simulink model "AGTF30SysDyn"  (Simulink 8.5)
settings: Solver=ode4  StartTime=0.0  StopTime=MWS.In.t(end)  FixedStep=MWS.In.Ts  RelTol=1e-3
model workspace: external: MAT-File (data not in the file)
values from neighbouring files (symbols this model uses):
  MWS = setup_InputsSS(MWS)    [define_inputs.m]
libraries: Lib_Cntrl_FirstOrderSensor_TMATS x12, Lib_Solve_ModelSource_TMATS x8, Lib_Cntrl_LimitCntrlPI_TMATS x5, Lib_Cntrl_FirstOrderActuator_TMATS x2, Lib_Cntrl_SetPoint_TMATS x2, Lib_Solve_OuterLoopIntegrator_TMATS x2, simulink x2, Lib_Cntrl_CorrectedSpeed_TMATS x1, Lib_Cntrl_LimitSelect_TMATS x1, Lib_Cntrl_SetPointCntrlPI_TMATS x1, Lib_Solve_IterNRSolverJC_TMATS x1
settings Model: Creator=jwchapm2  LastModifiedBy=jwchapm2
settings DataIOCC: SignalLoggingSaveFormat=Dataset
settings OptimizationCC: ExpressionDepthLimit=128
settings DebuggingCC: UnderspecifiedInitializationDetection=Simplified  MergeDetectMultiDrivingBlocksExec=error  FcnCallInpInsideContextMsg=EnableAllAsError  StateNameClashWarn=none
settings GRTTargetCC: CombineOutputUpdateFcns=on  GRTInterface=off

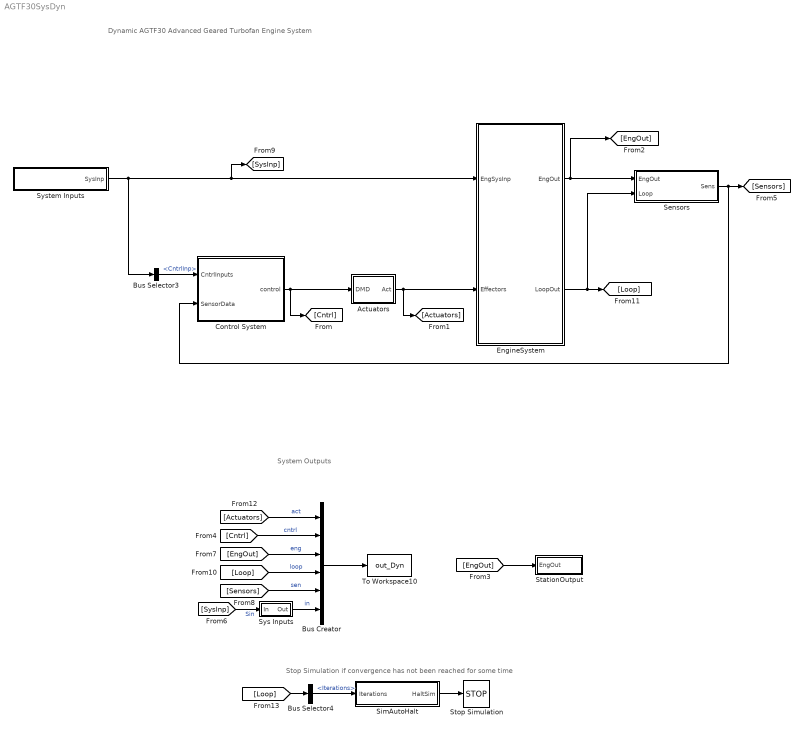
== system AGTF30SysDyn ==
  note: Stop Simulation if convergence has not been reached for some time
  note: Dynamic AGTF30
      | Advanced Geared Turbofan Engine System
  note: System Outputs
  Actuators : Subsystem
  Bus Creator : BusCreator  Inputs=6
  Bus Selector3 : BusSelector  OutputSignals=CntrlInp
  Bus Selector4 : BusSelector  OutputSignals=Solver.Iterations
  Control System : Subsystem
  EngineSystem : Subsystem
  Sensors : Subsystem
  SimAutoHalt : Subsystem
  StationOutput : Subsystem
  Stop Simulation : Stop
  Sys Inputs : Subsystem
  System Inputs : Subsystem
  To Workspace10 : ToWorkspace  VariableName=out_Dyn  SaveFormat=Timeseries  SampleTime=-1
  wires:
  Actuators/1(Act) -> [Actuators], EngineSystem/2(Effectors)
  Control System/1(control) -> Actuators/1(DMD), [Cntrl]
  Bus Selector3/1 -> Control System/1(CntrlInputs)  "<CntrlInp>"
  System Inputs/1(SysInp) -> Bus Selector3/1, EngineSystem/1(EngSysInp), [SysInp]
  EngineSystem/1(EngOut) -> [EngOut], Sensors/1(EngOut)
  EngineSystem/2(LoopOut) -> Sensors/2(Loop), [Loop]
  [EngOut] -> StationOutput/1(EngOut)
  Bus Creator/1 -> To Workspace10/1
  [Loop] -> Bus Creator/4  "loop"
  [Sensors] -> Bus Creator/5  "sen"
  [EngOut] -> Bus Creator/3  "eng"
  Sys Inputs/1(Out) -> Bus Creator/6  "in"
  [Actuators] -> Bus Creator/1  "act"
  [Cntrl] -> Bus Creator/2  "cntrl"
  Sensors/1(Sens) -> Control System/2(SensorData), [Sensors]
  [Loop] -> Bus Selector4/1
  Bus Selector4/1 -> SimAutoHalt/1(Iterations)  "<Iterations>"
  SimAutoHalt/1(HaltSim) -> Stop Simulation/1
  [SysInp] -> Sys Inputs/1(In)  "Sin"

== system AGTF30SysDyn/Actuators ==
  DMD : Inport
  Bus Creator : BusCreator  Inputs=3
  Bus Selector1 : BusSelector  OutputSignals=Wfdmd,VBVdmd,VAFNdmd
  FMV : Subsystem
  VAFN : Subsystem
  VBV : Subsystem
  Act : Outport
  wires:
  DMD/1 -> Bus Selector1/1
  Bus Creator/1 -> Act/1  "Actuator"
  Bus Selector1/3 -> VAFN/1(VAFNdmd)  "<VAFNdmd>"
  Bus Selector1/2 -> VBV/1(VBVdmd)  "<VBVdmd>"
  VBV/1(VBVact) -> Bus Creator/2  "VBVact"
  VAFN/1(VAFNact) -> Bus Creator/3  "VAFNact"
  Bus Selector1/1 -> FMV/1(Wfdmd)  "<Wfdmd>"
  FMV/1(Wfact) -> Bus Creator/1  "Wfact"

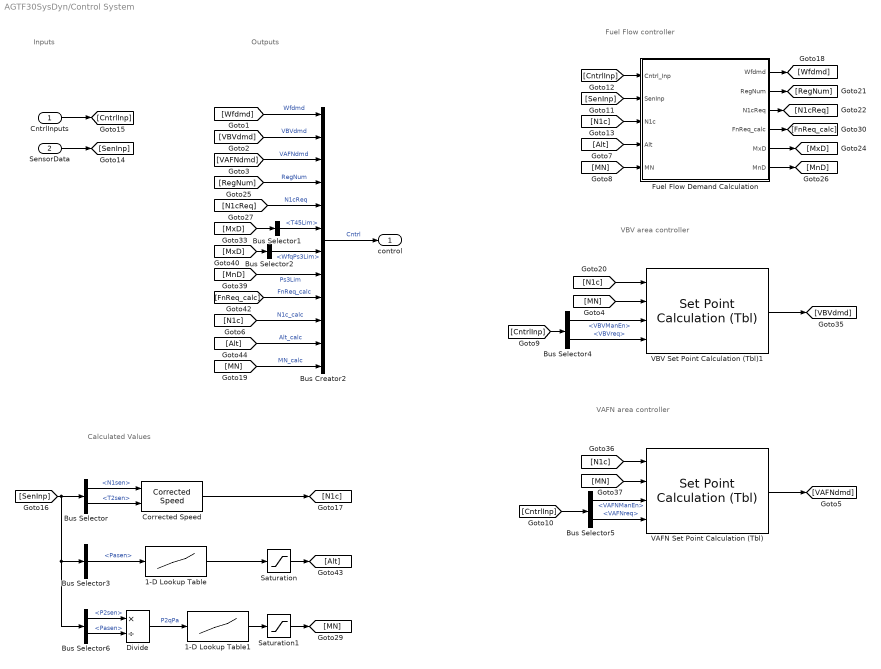
== system AGTF30SysDyn/Control System ==
  note: Inputs
  note: VAFN area controller
  note: VBV area controller
  note: Fuel Flow controller
  note: Calculated Values
  note: Outputs
  CntrlInputs : Inport
  SensorData : Inport  Port=2
  1-D Lookup Table : Lookup_n-D  NumberOfTableDimensions=1  BreakpointsForDimension1=MWS.Cntrl.AltCalc_PaVec  Table=MWS.Cntrl.AltCalc_AltVec  InternalRulePriority=Speed  RndMeth=Simplest  InputSameDT=on
  1-D Lookup Table1 : Lookup_n-D  NumberOfTableDimensions=1  BreakpointsForDimension1=MWS.Cntrl.MNCalc_P2qPa  Table=MWS.Cntrl.MNCalc_MNVec  InternalRulePriority=Speed  RndMeth=Simplest  InputSameDT=on
  Bus Creator2 : BusCreator  Inputs=12
  Bus Selector : BusSelector  OutputSignals=N.N1sen,T.T2sen
  Bus Selector1 : BusSelector  OutputSignals=T45Lim
  Bus Selector2 : BusSelector  OutputSignals=WfqPs3Lim
  Bus Selector3 : BusSelector  OutputSignals=P.Pasen
  Bus Selector4 : BusSelector  OutputSignals=ManualOp.VBVManEn,ManualOp.VBVreq
  Bus Selector5 : BusSelector  OutputSignals=ManualOp.VAFNManEn,ManualOp.VAFNreq
  Bus Selector6 : BusSelector  OutputSignals=P.P2sen,P.Pasen
  Corrected Speed : Lib_Cntrl_CorrectedSpeed_TMATS/Corrected Speed  C_TSTD_M=518.67
  Divide : Product  Inputs=*/
  Fuel Flow Demand Calculation : Subsystem
  Saturation : Saturate  UpperLimit=MWS.Cntrl.AltCalc_Altmax  LowerLimit=MWS.Cntrl.AltCalc_Altmin
  Saturation1 : Saturate  UpperLimit=MWS.Cntrl.MNCalc_MNmax  LowerLimit=MWS.Cntrl.MNCalc_MNmin
  VAFN Set Point Calculation (Tbl) : Lib_Cntrl_SetPoint_TMATS/Set Point Calculation (Tbl)  ERVec_M=MWS.Cntrl.VAFN_Nc1  DSVec_M=MWS.Cntrl.VAFN_MN  SPArray_M=MWS.Cntrl.VAFN_sch
  VBV Set Point Calculation (Tbl)1 : Lib_Cntrl_SetPoint_TMATS/Set Point Calculation (Tbl)  ERVec_M=MWS.Cntrl.VBV_Nc1  DSVec_M=MWS.Cntrl.VBV_MN  SPArray_M=MWS.Cntrl.VBV_sch
  control : Outport
  wires:
  CntrlInputs/1 -> [CntrlInp]
  [Wfdmd] -> Bus Creator2/1  "Wfdmd"
  [VBVdmd] -> Bus Creator2/2  "VBVdmd"
  [VAFNdmd] -> Bus Creator2/3  "VAFNdmd"
  SensorData/1 -> [SenInp]
  Bus Selector/1 -> Corrected Speed/1  "<N1sen>"
  Corrected Speed/1 -> [N1c]
  Bus Selector/2 -> Corrected Speed/2  "<T2sen>"
  [CntrlInp] -> Bus Selector4/1
  [RegNum] -> Bus Creator2/4  "RegNum"
  VAFN Set Point Calculation (Tbl)/1 -> [VAFNdmd]
  [CntrlInp] -> Bus Selector5/1
  Bus Selector4/1 -> VBV Set Point Calculation (Tbl)1/3  "<VBVManEn>"
  Bus Selector4/2 -> VBV Set Point Calculation (Tbl)1/4  "<VBVreq>"
  [MN] -> VBV Set Point Calculation (Tbl)1/2
  VBV Set Point Calculation (Tbl)1/1 -> [VBVdmd]
  Bus Selector5/2 -> VAFN Set Point Calculation (Tbl)/4  "<VAFNreq>"
  Bus Selector5/1 -> VAFN Set Point Calculation (Tbl)/3  "<VAFNManEn>"
  [MN] -> VAFN Set Point Calculation (Tbl)/2
  [N1c] -> VAFN Set Point Calculation (Tbl)/1
  [N1c] -> VBV Set Point Calculation (Tbl)1/1
  [N1c] -> Bus Creator2/10  "N1c_calc"
  [N1cReq] -> Bus Creator2/5  "N1cReq"
  Bus Selector1/1 -> Bus Creator2/6  "<T45Lim>"
  [MxD] -> Bus Selector1/1
  [MnD] -> Bus Creator2/8  "Ps3Lim"
  [MxD] -> Bus Selector2/1
  Bus Selector2/1 -> Bus Creator2/7  "<WfqPs3Lim>"
  [FnReq_calc] -> Bus Creator2/9  "FnReq_calc"
  1-D Lookup Table/1 -> Saturation/1
  [SenInp] -> Bus Selector6/1, Bus Selector3/1, Bus Selector/1
  Bus Selector3/1 -> 1-D Lookup Table/1  "<Pasen>"
  Bus Selector6/1 -> Divide/1  "<P2sen>"
  Bus Selector6/2 -> Divide/2  "<Pasen>"
  Divide/1 -> 1-D Lookup Table1/1  "P2qPa"
  1-D Lookup Table1/1 -> Saturation1/1
  [Alt] -> Bus Creator2/11  "Alt_calc"
  [MN] -> Bus Creator2/12  "MN_calc"
  Saturation/1 -> [Alt]
  Saturation1/1 -> [MN]
  Bus Creator2/1 -> control/1  "Cntrl"
  [CntrlInp] -> Fuel Flow Demand Calculation/1(Cntrl_Inp)
  [Alt] -> Fuel Flow Demand Calculation/4("Alt ")
  [MN] -> Fuel Flow Demand Calculation/5(MN)
  [SenInp] -> Fuel Flow Demand Calculation/2(SenInp)
  [N1c] -> Fuel Flow Demand Calculation/3(N1c)
  Fuel Flow Demand Calculation/6(MnD) -> [MnD]
  Fuel Flow Demand Calculation/5(MxD) -> [MxD]
  Fuel Flow Demand Calculation/4(FnReq_calc) -> [FnReq_calc]
  Fuel Flow Demand Calculation/3(N1cReq) -> [N1cReq]
  Fuel Flow Demand Calculation/2(RegNum) -> [RegNum]
  Fuel Flow Demand Calculation/1(Wfdmd) -> [Wfdmd]

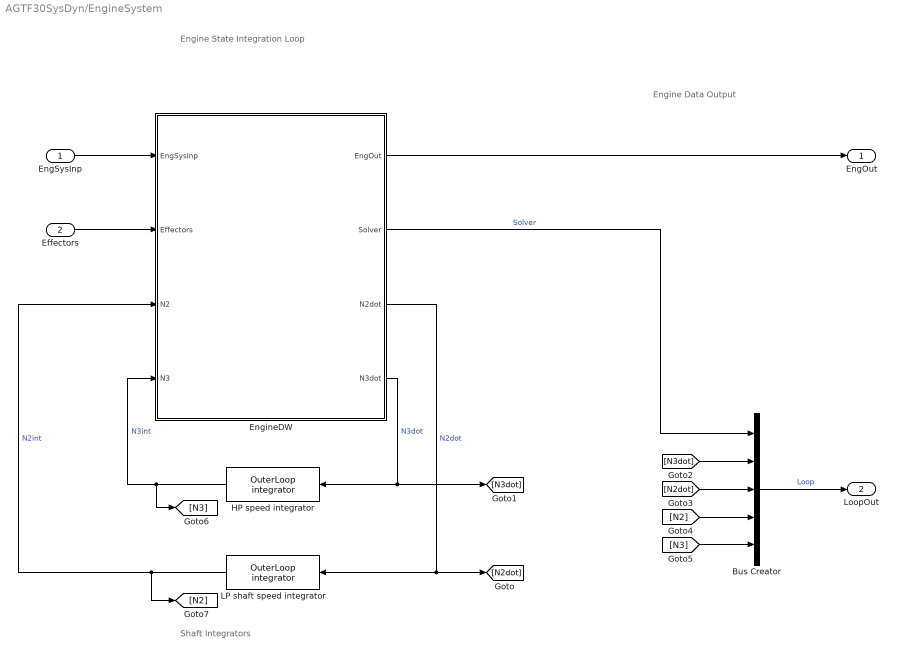
== system AGTF30SysDyn/EngineSystem ==
  note: Shaft Integrators
  note: Engine State
      | Integration Loop
  note: Engine Data Output
  EngSysInp : Inport
  Effectors : Inport  Port=2
  Bus Creator : BusCreator  Inputs=5
  EngineDW : Subsystem
  HP speed integrator : Lib_Solve_OuterLoopIntegrator_TMATS/OuterLoop integrator  OL_IC_M=MWS.In.N3IC
  LP shaft speed integrator : Lib_Solve_OuterLoopIntegrator_TMATS/OuterLoop integrator  OL_IC_M=MWS.In.N2IC
  EngOut : Outport
  LoopOut : Outport  Port=2
  wires:
  EngSysInp/1 -> EngineDW/1(EngSysInp)
  LP shaft speed integrator/1 -> [N2], EngineDW/3(N2)  "N2int"
  Effectors/1 -> EngineDW/2(Effectors)
  EngineDW/3(N2dot) -> LP shaft speed integrator/1, [N2dot]  "N2dot"
  EngineDW/2(Solver) -> Bus Creator/1  "Solver"
  EngineDW/1(EngOut) -> EngOut/1
  EngineDW/4(N3dot) -> HP speed integrator/1, [N3dot]  "N3dot"
  HP speed integrator/1 -> [N3], EngineDW/4(N3)  "N3int"
  Bus Creator/1 -> LoopOut/1  "Loop"
  [N3dot] -> Bus Creator/2
  [N2dot] -> Bus Creator/3
  [N2] -> Bus Creator/4
  [N3] -> Bus Creator/5

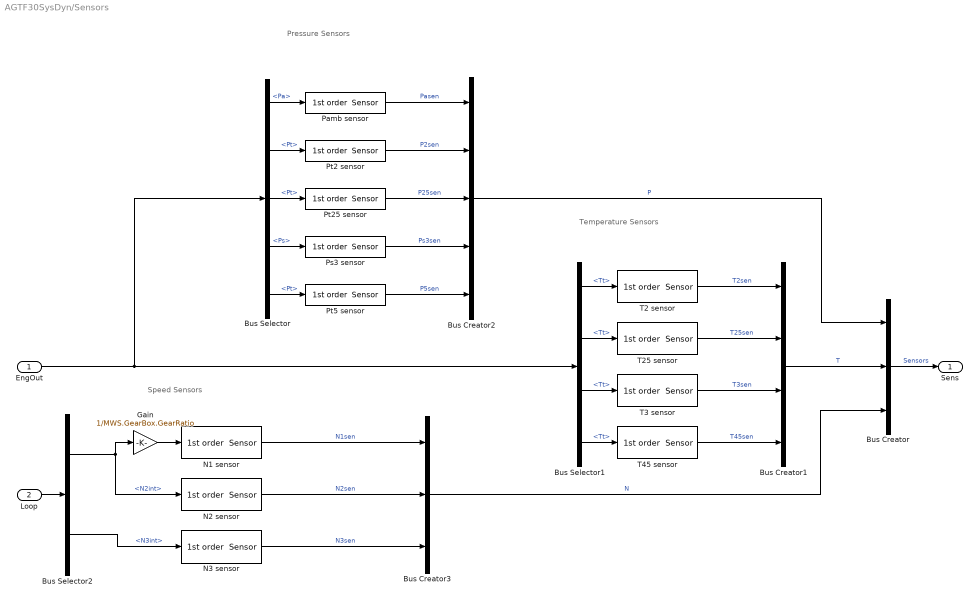
== system AGTF30SysDyn/Sensors ==
  note: Pressure Sensors
  note: Temperature Sensors
  note: Speed Sensors
  EngOut : Inport
  Loop : Inport  Port=2
  Bus Creator : BusCreator  Inputs=3
  Bus Creator1 : BusCreator
  Bus Creator2 : BusCreator  Inputs=5
  Bus Creator3 : BusCreator  Inputs=3
  Bus Selector : BusSelector  OutputSignals=Amb.Pa,S2.Pt,S25.Pt,S36.Ps,S5.Pt
  Bus Selector1 : BusSelector  OutputSignals=S2.Tt,S25.Tt,S36.Tt,S45.Tt
  Bus Selector2 : BusSelector  OutputSignals=N2int,N3int
  Gain : Gain  Gain=1/MWS.GearBox.GearRatio
  N1 sensor : Lib_Cntrl_FirstOrderSensor_TMATS/1st order  Sensor  IC_M=MWS.In.Sensor.ICN1  Sen_Max_M=MWS.Sensor.N1.Max  Sen_Min_M=MWS.Sensor.N1.Min  Gain_M=1  Tau_M=MWS.Sensor.N1.Tau  GN_EN_M=off  GN_NST_M=MWS.In.Ts  GN_C_M=1  GN_MinNoise_M=0.3  F_Gain_M=1  F_Drift_M=0
  N2 sensor : Lib_Cntrl_FirstOrderSensor_TMATS/1st order  Sensor  IC_M=MWS.In.Sensor.ICN2  Sen_Max_M=MWS.Sensor.N2.Max  Sen_Min_M=MWS.Sensor.N2.Min  Gain_M=1  Tau_M=MWS.Sensor.N2.Tau  GN_EN_M=off  GN_NST_M=MWS.In.Ts  GN_C_M=1  GN_MinNoise_M=0.3  F_Gain_M=1  F_Drift_M=0
  N3 sensor : Lib_Cntrl_FirstOrderSensor_TMATS/1st order  Sensor  IC_M=MWS.In.Sensor.ICN3  Sen_Max_M=MWS.Sensor.N3.Max  Sen_Min_M=MWS.Sensor.N3.Min  Gain_M=1  Tau_M=MWS.Sensor.N3.Tau  GN_EN_M=off  GN_NST_M=MWS.In.Ts  GN_C_M=1  GN_MinNoise_M=0.3  F_Gain_M=1  F_Drift_M=0
  Pamb sensor : Lib_Cntrl_FirstOrderSensor_TMATS/1st order  Sensor  IC_M=MWS.In.Sensor.ICPa  Sen_Max_M=MWS.Sensor.P2.Max  Sen_Min_M=MWS.Sensor.P2.Min  Gain_M=1  Tau_M=MWS.Sensor.P2.Tau  GN_EN_M=off  GN_NST_M=MWS.In.Ts  GN_C_M=1  GN_MinNoise_M=0.3  F_Gain_M=1  F_Drift_M=0
  Ps3 sensor : Lib_Cntrl_FirstOrderSensor_TMATS/1st order  Sensor  IC_M=MWS.In.Sensor.ICPs3  Sen_Max_M=MWS.Sensor.Ps3.Max  Sen_Min_M=MWS.Sensor.Ps3.Min  Gain_M=1  Tau_M=MWS.Sensor.Ps3.Tau  GN_EN_M=off  GN_NST_M=MWS.In.Ts  GN_C_M=1  GN_MinNoise_M=0.3  F_Gain_M=1  F_Drift_M=0
  Pt2 sensor : Lib_Cntrl_FirstOrderSensor_TMATS/1st order  Sensor  IC_M=MWS.In.Sensor.ICP2  Sen_Max_M=MWS.Sensor.P2.Max  Sen_Min_M=MWS.Sensor.P2.Min  Gain_M=1  Tau_M=MWS.Sensor.P2.Tau  GN_EN_M=off  GN_NST_M=MWS.In.Ts  GN_C_M=1  GN_MinNoise_M=0.3  F_Gain_M=1  F_Drift_M=0
  Pt25 sensor : Lib_Cntrl_FirstOrderSensor_TMATS/1st order  Sensor  IC_M=MWS.In.Sensor.ICP25  Sen_Max_M=MWS.Sensor.P25.Max  Sen_Min_M=MWS.Sensor.P25.Min  Gain_M=1  Tau_M=MWS.Sensor.P25.Tau  GN_EN_M=off  GN_NST_M=MWS.In.Ts  GN_C_M=1  GN_MinNoise_M=0.3  F_Gain_M=1  F_Drift_M=0
  Pt5 sensor : Lib_Cntrl_FirstOrderSensor_TMATS/1st order  Sensor  IC_M=MWS.In.Sensor.ICP5  Sen_Max_M=MWS.Sensor.P5.Max  Sen_Min_M=MWS.Sensor.P5.Min  Gain_M=1  Tau_M=MWS.Sensor.P5.Tau  GN_EN_M=off  GN_NST_M=MWS.In.Ts  GN_C_M=1  GN_MinNoise_M=0.3  F_Gain_M=1  F_Drift_M=0
  T2 sensor : Lib_Cntrl_FirstOrderSensor_TMATS/1st order  Sensor  IC_M=MWS.In.Sensor.ICT2  Sen_Max_M=MWS.Sensor.T2.Max  Sen_Min_M=MWS.Sensor.T2.Min  Gain_M=1  Tau_M=MWS.Sensor.T2.Tau  GN_EN_M=off  GN_NST_M=MWS.In.Ts  GN_C_M=1  GN_MinNoise_M=0.3  F_Gain_M=1  F_Drift_M=0
  T25 sensor : Lib_Cntrl_FirstOrderSensor_TMATS/1st order  Sensor  IC_M=MWS.In.Sensor.ICT25  Sen_Max_M=MWS.Sensor.T25.Max  Sen_Min_M=MWS.Sensor.T25.Min  Gain_M=1  Tau_M=MWS.Sensor.T25.Tau  GN_EN_M=off  GN_NST_M=MWS.In.Ts  GN_C_M=1  GN_MinNoise_M=0.3  F_Gain_M=1  F_Drift_M=0
  T3 sensor : Lib_Cntrl_FirstOrderSensor_TMATS/1st order  Sensor  IC_M=MWS.In.Sensor.ICT3  Sen_Max_M=MWS.Sensor.T3.Max  Sen_Min_M=MWS.Sensor.T3.Min  Gain_M=1  Tau_M=MWS.Sensor.T3.Tau  GN_EN_M=off  GN_NST_M=MWS.In.Ts  GN_C_M=1  GN_MinNoise_M=0.3  F_Gain_M=1  F_Drift_M=0
  T45 sensor : Lib_Cntrl_FirstOrderSensor_TMATS/1st order  Sensor  IC_M=MWS.In.Sensor.ICT45  Sen_Max_M=MWS.Sensor.T45.Max*10  Sen_Min_M=MWS.Sensor.T45.Min  Gain_M=1  Tau_M=MWS.Sensor.T45.Tau  GN_EN_M=off  GN_NST_M=MWS.In.Ts  GN_C_M=1  GN_MinNoise_M=0.3  F_Gain_M=1  F_Drift_M=0
  Sens : Outport
  wires:
  Bus Creator/1 -> Sens/1  "Sensors"
  Bus Selector/2 -> Pt2 sensor/1  "<Pt>"
  Bus Creator2/1 -> Bus Creator/1  "P"
  Bus Creator1/1 -> Bus Creator/2  "T"
  Bus Selector1/1 -> T2 sensor/1  "<Tt>"
  Bus Creator3/1 -> Bus Creator/3  "N"
  Bus Selector/3 -> Pt25 sensor/1  "<Pt>"
  Bus Selector/5 -> Pt5 sensor/1  "<Pt>"
  Pt2 sensor/1 -> Bus Creator2/2  "P2sen"
  Pt25 sensor/1 -> Bus Creator2/3  "P25sen"
  Pt5 sensor/1 -> Bus Creator2/5  "P5sen"
  Bus Selector1/2 -> T25 sensor/1  "<Tt>"
  Bus Selector1/3 -> T3 sensor/1  "<Tt>"
  Bus Selector1/4 -> T45 sensor/1  "<Tt>"
  T2 sensor/1 -> Bus Creator1/1  "T2sen"
  T25 sensor/1 -> Bus Creator1/2  "T25sen"
  T3 sensor/1 -> Bus Creator1/3  "T3sen"
  N1 sensor/1 -> Bus Creator3/1  "N1sen"
  Bus Selector/4 -> Ps3 sensor/1  "<Ps>"
  N3 sensor/1 -> Bus Creator3/3  "N3sen"
  Bus Selector/1 -> Pamb sensor/1  "<Pa>"
  Pamb sensor/1 -> Bus Creator2/1  "Pasen"
  N2 sensor/1 -> Bus Creator3/2  "N2sen"
  EngOut/1 -> Bus Selector/1, Bus Selector1/1
  Bus Selector2/2 -> N3 sensor/1  "<N3int>"
  Bus Selector2/1 -> N2 sensor/1, Gain/1  "<N2int>"
  Gain/1 -> N1 sensor/1
  Loop/1 -> Bus Selector2/1
  T45 sensor/1 -> Bus Creator1/4  "T45sen"
  Ps3 sensor/1 -> Bus Creator2/4  "Ps3sen"

== system AGTF30SysDyn/SimAutoHalt ==
  Iterations : Inport
  Compare To Constant : simulink/Logic and Bit Operations/Compare To Constant  relop=>=  const=MWS.In.Max_IterDyn  OutDataTypeStr=boolean
  Compare To Constant1 : simulink/Logic and Bit Operations/Compare To Constant  relop=>=  const=MWS.In.DynRunNonConv  OutDataTypeStr=boolean
  Constant : Constant
  Product : Product
  Sum : Sum  Inputs=|++
  Unit Delay : UnitDelay  SampleTime=-1
  HaltSim : Outport
  wires:
  Compare To Constant1/1 -> HaltSim/1
  Iterations/1 -> Compare To Constant/1
  Compare To Constant/1 -> Product/1
  Constant/1 -> Sum/1
  Sum/1 -> Unit Delay/1
  Unit Delay/1 -> Product/2
  Product/1 -> Sum/2, Compare To Constant1/1

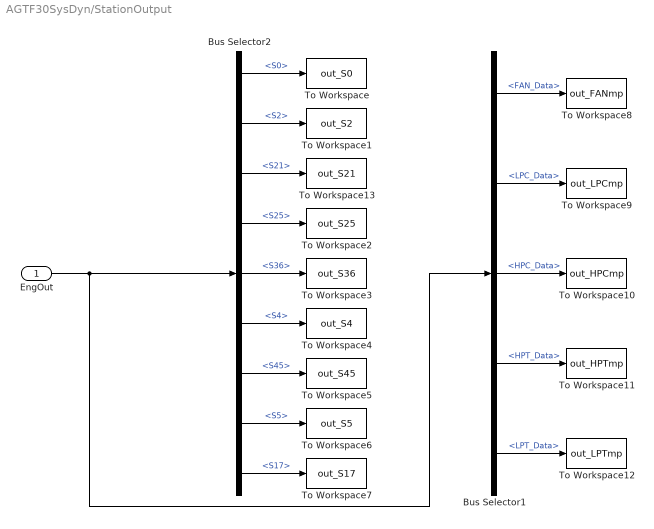
== system AGTF30SysDyn/StationOutput ==
  EngOut : Inport
  Bus Selector1 : BusSelector  OutputSignals=Data.FAN_Data,Data.LPC_Data,Data.HPC_Data,Data.HPT_Data,Data.LPT_Data
  Bus Selector2 : BusSelector  OutputSignals=S0,S2,S21,S25,S36,S4,S45,S5,S17
  To Workspace : ToWorkspace  VariableName=out_S0  SaveFormat=Timeseries  SampleTime=-1
  To Workspace1 : ToWorkspace  VariableName=out_S2  SaveFormat=Timeseries  SampleTime=-1
  To Workspace10 : ToWorkspace  VariableName=out_HPCmp  SaveFormat=Timeseries  SampleTime=-1
  To Workspace11 : ToWorkspace  VariableName=out_HPTmp  SaveFormat=Timeseries  SampleTime=-1
  To Workspace12 : ToWorkspace  VariableName=out_LPTmp  SaveFormat=Timeseries  SampleTime=-1
  To Workspace13 : ToWorkspace  VariableName=out_S21  SaveFormat=Timeseries  SampleTime=-1
  To Workspace2 : ToWorkspace  VariableName=out_S25  SaveFormat=Timeseries  SampleTime=-1
  To Workspace3 : ToWorkspace  VariableName=out_S36  SaveFormat=Timeseries  SampleTime=-1
  To Workspace4 : ToWorkspace  VariableName=out_S4  SaveFormat=Timeseries  SampleTime=-1
  To Workspace5 : ToWorkspace  VariableName=out_S45  SaveFormat=Timeseries  SampleTime=-1
  To Workspace6 : ToWorkspace  VariableName=out_S5  SaveFormat=Timeseries  SampleTime=-1
  To Workspace7 : ToWorkspace  VariableName=out_S17  SaveFormat=Timeseries  SampleTime=-1
  To Workspace8 : ToWorkspace  VariableName=out_FANmp  SaveFormat=Timeseries  SampleTime=-1
  To Workspace9 : ToWorkspace  VariableName=out_LPCmp  SaveFormat=Timeseries  SampleTime=-1
  wires:
  Bus Selector2/3 -> To Workspace13/1  "<S21>"
  Bus Selector2/1 -> To Workspace/1  "<S0>"
  EngOut/1 -> Bus Selector1/1, Bus Selector2/1
  Bus Selector2/2 -> To Workspace1/1  "<S2>"
  Bus Selector2/4 -> To Workspace2/1  "<S25>"
  Bus Selector2/5 -> To Workspace3/1  "<S36>"
  Bus Selector2/6 -> To Workspace4/1  "<S4>"
  Bus Selector2/7 -> To Workspace5/1  "<S45>"
  Bus Selector2/8 -> To Workspace6/1  "<S5>"
  Bus Selector2/9 -> To Workspace7/1  "<S17>"
  Bus Selector1/1 -> To Workspace8/1  "<FAN_Data>"
  Bus Selector1/2 -> To Workspace9/1  "<LPC_Data>"
  Bus Selector1/3 -> To Workspace10/1  "<HPC_Data>"
  Bus Selector1/4 -> To Workspace11/1  "<HPT_Data>"
  Bus Selector1/5 -> To Workspace12/1  "<LPT_Data>"

== system AGTF30SysDyn/Sys Inputs ==
  In : Inport
  Bus Creator1 : BusCreator  Inputs=12
  Bus Selector : BusSelector  OutputSignals=Env.Alt,Env.dT,Env.MN,CntrlInp.PLA,CntrlInp.ManualOp.WfMan,CntrlInp.ManualOp.WfManEn,CntrlInp.ManualOp.N1cMan,CntrlInp.ManualOp.N1ManEn,CntrlInp.ManualOp.VBVreq,CntrlInp.ManualOp.VBVManEn,CntrlInp.ManualOp.VAFNreq,CntrlInp.ManualOp.VAFNManEn
  Out : Outport
  wires:
  In/1 -> Bus Selector/1
  Bus Selector/4 -> Bus Creator1/4  "<PLA>"
  Bus Selector/6 -> Bus Creator1/6  "<WfManEn>"
  Bus Selector/7 -> Bus Creator1/7  "<N1cMan>"
  Bus Selector/8 -> Bus Creator1/8  "<N1ManEn>"
  Bus Selector/9 -> Bus Creator1/9  "<VBVreq>"
  Bus Selector/10 -> Bus Creator1/10  "<VBVManEn>"
  Bus Selector/11 -> Bus Creator1/11  "<VAFNreq>"
  Bus Selector/3 -> Bus Creator1/3  "<MN>"
  Bus Selector/5 -> Bus Creator1/5  "<WfMan>"
  Bus Selector/1 -> Bus Creator1/1  "<Alt>"
  Bus Selector/12 -> Bus Creator1/12  "<VAFNManEn>"
  Bus Selector/2 -> Bus Creator1/2  "<dT>"
  Bus Creator1/1 -> Out/1

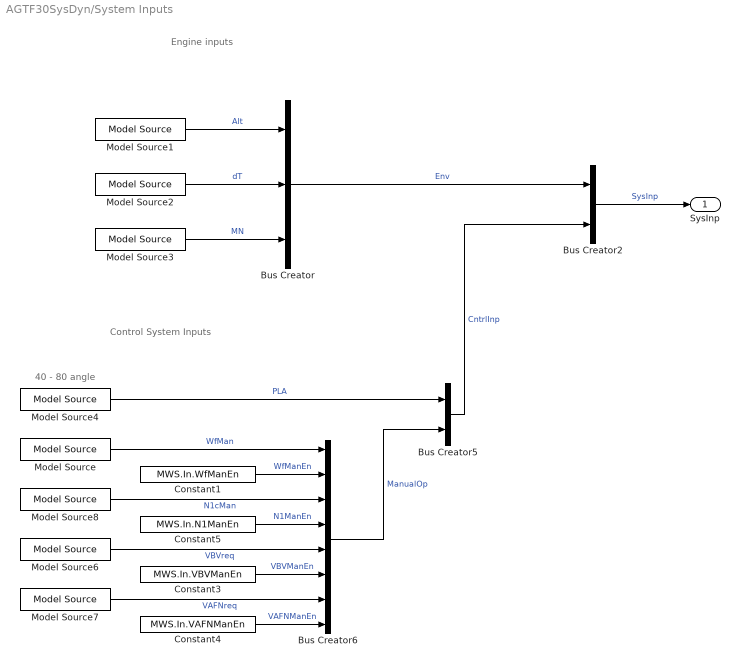
== system AGTF30SysDyn/System Inputs ==
  note: Engine inputs
  note: Control System Inputs
  note: 40 - 80 angle
  Bus Creator : BusCreator  Inputs=3
  Bus Creator2 : BusCreator  Inputs=2
  Bus Creator5 : BusCreator  Inputs=2
  Bus Creator6 : BusCreator  Inputs=8
  Constant1 : Constant  Value=MWS.In.WfManEn
  Constant3 : Constant  Value=MWS.In.VBVManEn
  Constant4 : Constant  Value=MWS.In.VAFNManEn
  Constant5 : Constant  Value=MWS.In.N1ManEn
  Model Source : Lib_Solve_ModelSource_TMATS/Model Source  T_vec_M=MWS.In.Wfreq(2,:)  input_array_M=MWS.In.Wfreq(1,:)
  Model Source1 : Lib_Solve_ModelSource_TMATS/Model Source  T_vec_M=MWS.In.Alt(2,:)  input_array_M=MWS.In.Alt(1,:)
  Model Source2 : Lib_Solve_ModelSource_TMATS/Model Source  T_vec_M=MWS.In.dT(2,:)  input_array_M=MWS.In.dT(1,:)
  Model Source3 : Lib_Solve_ModelSource_TMATS/Model Source  T_vec_M=MWS.In.MN(2,:)  input_array_M=MWS.In.MN(1,:)
  Model Source4 : Lib_Solve_ModelSource_TMATS/Model Source  T_vec_M=MWS.In.PLA(2,:)  input_array_M=MWS.In.PLA(1,:)
  Model Source6 : Lib_Solve_ModelSource_TMATS/Model Source  T_vec_M=MWS.In.VBVreq(2,:)  input_array_M=MWS.In.VBVreq(1,:)
  Model Source7 : Lib_Solve_ModelSource_TMATS/Model Source  T_vec_M=MWS.In.VAFNreq(2,:)  input_array_M=MWS.In.VAFNreq(1,:)
  Model Source8 : Lib_Solve_ModelSource_TMATS/Model Source  T_vec_M=MWS.In.N1creq(2,:)  input_array_M=MWS.In.N1creq(1,:)
  SysInp : Outport
  wires:
  Model Source1/1 -> Bus Creator/1  "Alt"
  Model Source2/1 -> Bus Creator/2  "dT"
  Model Source3/1 -> Bus Creator/3  "MN"
  Bus Creator/1 -> Bus Creator2/1  "Env"
  Bus Creator5/1 -> Bus Creator2/2  "CntrlInp"
  Bus Creator2/1 -> SysInp/1  "SysInp"
  Model Source6/1 -> Bus Creator6/5  "VBVreq"
  Model Source7/1 -> Bus Creator6/7  "VAFNreq"
  Model Source4/1 -> Bus Creator5/1  "PLA"
  Bus Creator6/1 -> Bus Creator5/2  "ManualOp"
  Model Source/1 -> Bus Creator6/1  "WfMan"
  Constant1/1 -> Bus Creator6/2  "WfManEn"
  Constant4/1 -> Bus Creator6/8  "VAFNManEn"
  Constant3/1 -> Bus Creator6/6  "VBVManEn"
  Model Source8/1 -> Bus Creator6/3  "N1cMan"
  Constant5/1 -> Bus Creator6/4  "N1ManEn"

== system AGTF30SysDyn/Actuators/FMV ==
  Wfdmd : Inport
  1st order Actuator : Lib_Cntrl_FirstOrderActuator_TMATS/1st order Actuator  Gain_M=MWS.Act.FMV.Gain  Tau_M=MWS.Act.FMV.Tau  IC_M=MWS.In.WfIC  MaxSat_M=MWS.Act.FMV.max  MinSat_M=MWS.Act.FMV.min  deadband_M=0.0  rateLimit_M=MWS.Act.FMV.rateLimit
  Wf delay : TransportDelay  DelayTime=MWS.Act.FMV.TWf_dly  InitialOutput=MWS.In.WfIC
  Wfact : Outport
  wires:
  Wf delay/1 -> Wfact/1  "Wfact"
  Wfdmd/1 -> 1st order Actuator/1
  1st order Actuator/1 -> Wf delay/1

== system AGTF30SysDyn/Actuators/VAFN ==
  VAFNdmd : Inport
  Saturation1 : Saturate  UpperLimit=MWS.Act.VAFN_max  LowerLimit=0  LinearizeAsGain=off
  VAFN Dynamics : StateSpace  A=MWS.Act.VAFN.A  B=MWS.Act.VAFN.B  C=MWS.Act.VAFN.C  D=MWS.Act.VAFN.D  X0=MWS.In.VAFNIC
  VAFNact : Outport
  wires:
  Saturation1/1 -> VAFNact/1
  VAFNdmd/1 -> VAFN Dynamics/1
  VAFN Dynamics/1 -> Saturation1/1

== system AGTF30SysDyn/Actuators/VBV ==
  VBVdmd : Inport
  1st order Actuator : Lib_Cntrl_FirstOrderActuator_TMATS/1st order Actuator  Gain_M=MWS.Act.VBV.Gain  Tau_M=MWS.Act.VBV.Tau  IC_M=MWS.In.VBVIC  MaxSat_M=MWS.Act.VBV.max  MinSat_M=MWS.Act.VBV.min  deadband_M=0.0  rateLimit_M=100000
  VBVact : Outport
  wires:
  VBVdmd/1 -> 1st order Actuator/1
  1st order Actuator/1 -> VBVact/1  "VBVact"

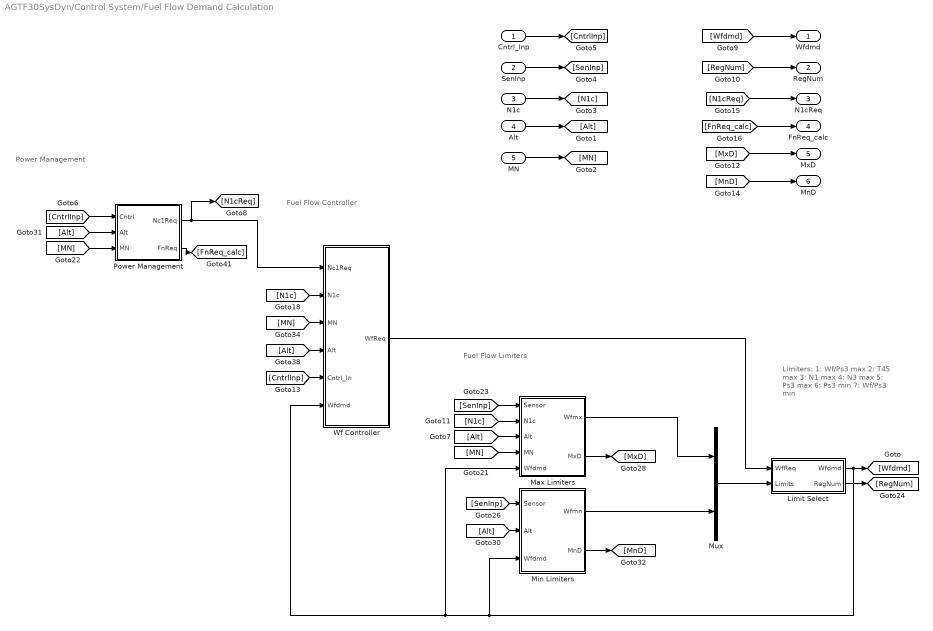
== system AGTF30SysDyn/Control System/Fuel Flow Demand Calculation ==
  note: Limiters:
      | 1: Wf/Ps3 max
      | 2: T45 max
      | 3: N1 max
      | 4: N3 max
      | 5: Ps3 max
      | 6: Ps3 min
      | 7: Wf/Ps3 min
  note: Fuel Flow Limiters
  note: Power Management
  note: Fuel Flow Controller
  Cntrl_Inp : Inport
  SenInp : Inport  Port=2
  N1c : Inport  Port=3
  "Alt " : Inport  Port=4
  MN : Inport  Port=5
  Limit Select : Subsystem
  Max Limiters : Subsystem
  Min Limiters : Subsystem
  Mux : Mux  Inputs=2
  Power Management : Subsystem
  Wf Controller : Subsystem
  Wfdmd : Outport
  RegNum : Outport  Port=2
  N1cReq : Outport  Port=3
  FnReq_calc : Outport  Port=4
  MxD : Outport  Port=5
  MnD : Outport  Port=6
  wires:
  [CntrlInp] -> Power Management/1(Cntrl)
  [SenInp] -> Max Limiters/1(Sensor)
  Max Limiters/1(Wfmx) -> Mux/1
  [MN] -> Max Limiters/4(MN)
  [MN] -> Wf Controller/3(MN)
  [Alt] -> Wf Controller/4(Alt)
  [CntrlInp] -> Wf Controller/5(Cntrl_In)
  Power Management/1(Nc1Req) -> Wf Controller/1(Nc1Req), [N1cReq]
  Min Limiters/1(Wfmn) -> Mux/2
  [Alt] -> Min Limiters/2(Alt)
  [SenInp] -> Min Limiters/1(Sensor)
  Limit Select/1(Wfdmd) -> [Wfdmd], Wf Controller/6(Wfdmd), Max Limiters/5(Wfdmd), Min Limiters/3("Wfdmd ")
  Wf Controller/1(WfReq) -> Limit Select/1(WfReq)
  Mux/1 -> Limit Select/2(Limits)
  Limit Select/2(RegNum) -> [RegNum]
  [N1c] -> Max Limiters/2(N1c)
  [Alt] -> Max Limiters/3(Alt)
  [MN] -> Power Management/3(MN)
  [Alt] -> Power Management/2(Alt)
  [N1c] -> Wf Controller/2(N1c)
  Max Limiters/2(MxD) -> [MxD]
  Min Limiters/2(MnD) -> [MnD]
  Power Management/2(FnReq) -> [FnReq_calc]
  "Alt "/1 -> [Alt]
  MN/1 -> [MN]
  N1c/1 -> [N1c]
  SenInp/1 -> [SenInp]
  Cntrl_Inp/1 -> [CntrlInp]
  [Wfdmd] -> Wfdmd/1
  [RegNum] -> RegNum/1
  [N1cReq] -> N1cReq/1
  [FnReq_calc] -> FnReq_calc/1
  [MxD] -> MxD/1
  [MnD] -> MnD/1

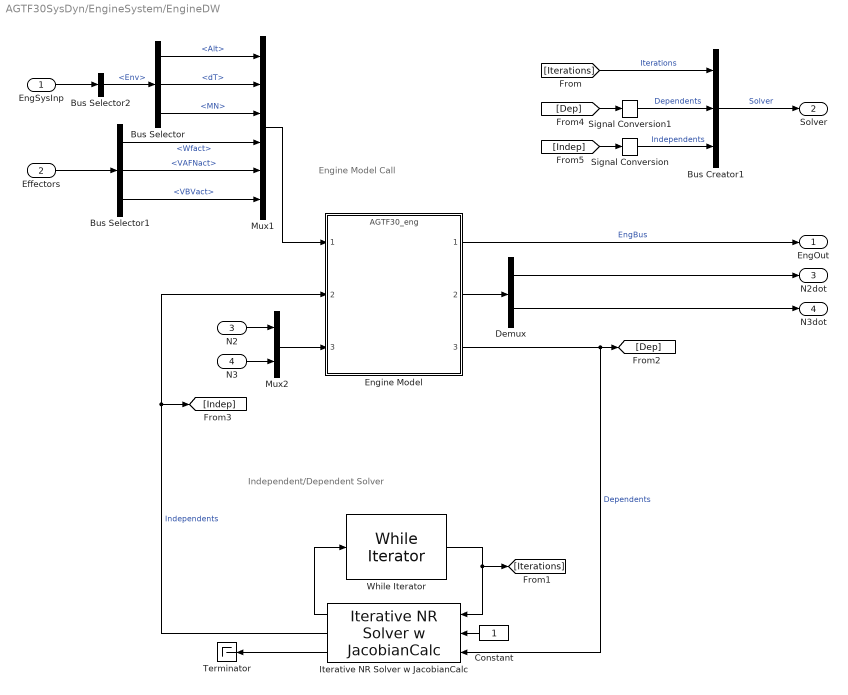
== system AGTF30SysDyn/EngineSystem/EngineDW ==
  note: Independent/Dependent Solver
  note: Engine Model Call
  EngSysInp : Inport
  Effectors : Inport  Port=2
  N2 : Inport  Port=3
  N3 : Inport  Port=4
  Bus Creator1 : BusCreator  Inputs=3
  Bus Selector : BusSelector  OutputSignals=Alt,dT,MN
  Bus Selector1 : BusSelector  OutputSignals=Wfact,VAFNact,VBVact
  Bus Selector2 : BusSelector  OutputSignals=Env
  Constant : Constant
  Demux : Demux  Outputs=2
  Engine Model : ModelReference  ModelNameDialog=AGTF30_eng.mdl  SimulationMode=Normal  ModelReferenceVersion=1.306  CopyOfModelName=AGTF30_eng.mdl  DefaultDataLogging=on
  Iterative NR Solver w JacobianCalc : Lib_Solve_IterNRSolverJC_TMATS/Iterative NR Solver w JacobianCalc  SJac_Per_M=MWS.In.JPerDyn  SNR_IC_M=MWS.In.ICcom  SNR_DX_M=MWS.In.dX  SNR_Mx_M=100000  SNR_Mn_M=0.0001  SJacobianAttempts_M=MWS.In.NRADyn  Cond_Limits_M=MWS.In.Lim
  Mux1 : Mux  Inputs=6
  Mux2 : Mux  Inputs=2
  Signal Conversion : SignalConversion
  Signal Conversion1 : SignalConversion
  Terminator : Terminator
  While Iterator : WhileIterator  MaxIters=MWS.In.Max_IterDyn  WhileBlockType=do-while  ShowIterationPort=on
  EngOut : Outport
  Solver : Outport  Port=2
  N2dot : Outport  Port=3
  N3dot : Outport  Port=4
  wires:
  Engine Model/1 -> EngOut/1  "EngBus"
  Mux1/1 -> Engine Model/1
  EngSysInp/1 -> Bus Selector2/1
  Effectors/1 -> Bus Selector1/1
  Constant/1 -> Iterative NR Solver w JacobianCalc/2
  Iterative NR Solver w JacobianCalc/2 -> Engine Model/2, [Indep]  "Independents"
  Engine Model/3 -> Iterative NR Solver w JacobianCalc/3, [Dep]  "Dependents"
  While Iterator/1 -> [Iterations], Iterative NR Solver w JacobianCalc/1
  Iterative NR Solver w JacobianCalc/1 -> While Iterator/1
  Engine Model/2 -> Demux/1
  Mux2/1 -> Engine Model/3
  Iterative NR Solver w JacobianCalc/3 -> Terminator/1
  N2/1 -> Mux2/1
  N3/1 -> Mux2/2
  Demux/1 -> N2dot/1
  Demux/2 -> N3dot/1
  Bus Selector/1 -> Mux1/1  "<Alt>"
  Bus Selector/2 -> Mux1/2  "<dT>"
  Bus Selector/3 -> Mux1/3  "<MN>"
  Bus Selector1/3 -> Mux1/6  "<VBVact>"
  Bus Selector1/1 -> Mux1/4  "<Wfact>"
  [Iterations] -> Bus Creator1/1  "Iterations"
  Bus Creator1/1 -> Solver/1  "Solver"
  [Dep] -> Signal Conversion1/1
  [Indep] -> Signal Conversion/1
  Signal Conversion/1 -> Bus Creator1/3  "Independents"
  Signal Conversion1/1 -> Bus Creator1/2  "Dependents"
  Bus Selector1/2 -> Mux1/5  "<VAFNact>"
  Bus Selector2/1 -> Bus Selector/1  "<Env>"

== system AGTF30SysDyn/Control System/Fuel Flow Demand Calculation/Limit Select ==
  WfReq : Inport
  Limits : Inport  Port=2
  Limit Selection : Lib_Cntrl_LimitSelect_TMATS/Limit Selection  SelectVec_M=MWS.Cntrl.Limit_Types  LimitsEn_M=MWS.Cntrl.Limit_En
  Wfdmd : Outport
  RegNum : Outport  Port=2
  wires:
  WfReq/1 -> Limit Selection/1
  Limits/1 -> Limit Selection/2
  Limit Selection/1 -> Wfdmd/1
  Limit Selection/2 -> RegNum/1

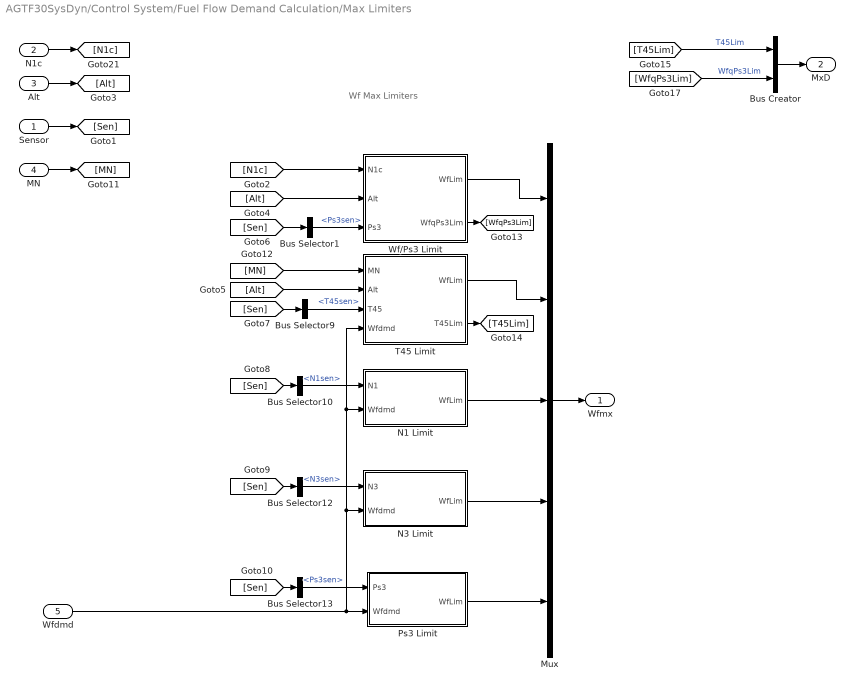
== system AGTF30SysDyn/Control System/Fuel Flow Demand Calculation/Max Limiters ==
  note: Wf Max Limiters
  Sensor : Inport
  N1c : Inport  Port=2
  Alt : Inport  Port=3
  MN : Inport  Port=4
  Wfdmd : Inport  Port=5
  Bus Creator : BusCreator  Inputs=2
  Bus Selector1 : BusSelector  OutputSignals=P.Ps3sen
  Bus Selector10 : BusSelector  OutputSignals=N.N1sen
  Bus Selector12 : BusSelector  OutputSignals=N.N3sen
  Bus Selector13 : BusSelector  OutputSignals=P.Ps3sen
  Bus Selector9 : BusSelector  OutputSignals=T.T45sen
  Mux : Mux  Inputs=5
  N1 Limit : Subsystem
  N3 Limit : Subsystem
  Ps3 Limit : Subsystem
  T45 Limit : Subsystem
  Wf/Ps3 Limit : Subsystem
  Wfmx : Outport
  MxD : Outport  Port=2
  wires:
  Wfdmd/1 -> T45 Limit/4(Wfdmd), N1 Limit/2(Wfdmd), N3 Limit/2(Wfdmd), Ps3 Limit/2(Wfdmd)
  Mux/1 -> Wfmx/1
  N1c/1 -> [N1c]
  Alt/1 -> [Alt]
  Wf/Ps3 Limit/1(WfLim) -> Mux/1
  [N1c] -> Wf/Ps3 Limit/1(N1c)
  [Alt] -> Wf/Ps3 Limit/2(Alt)
  Bus Selector1/1 -> Wf/Ps3 Limit/3(Ps3)  "<Ps3sen>"
  T45 Limit/1(WfLim) -> Mux/2
  [MN] -> T45 Limit/1(MN)
  [Alt] -> T45 Limit/2(Alt)
  Bus Selector9/1 -> T45 Limit/3(T45)  "<T45sen>"
  N1 Limit/1(WfLim) -> Mux/3
  Bus Selector10/1 -> N1 Limit/1(N1)  "<N1sen>"
  Bus Selector13/1 -> Ps3 Limit/1(Ps3)  "<Ps3sen>"
  Ps3 Limit/1(WfLim) -> Mux/5
  Bus Selector12/1 -> N3 Limit/1(N3)  "<N3sen>"
  N3 Limit/1(WfLim) -> Mux/4
  Sensor/1 -> [Sen]
  [Sen] -> Bus Selector1/1
  [Sen] -> Bus Selector9/1
  [Sen] -> Bus Selector10/1
  [Sen] -> Bus Selector12/1
  [Sen] -> Bus Selector13/1
  MN/1 -> [MN]
  Wf/Ps3 Limit/2(WfqPs3Lim) -> [WfqPs3Lim]
  T45 Limit/2(T45Lim) -> [T45Lim]
  [T45Lim] -> Bus Creator/1  "T45Lim"
  [WfqPs3Lim] -> Bus Creator/2  "WfqPs3Lim"
  Bus Creator/1 -> MxD/1

== system AGTF30SysDyn/Control System/Fuel Flow Demand Calculation/Min Limiters ==
  note: Wf Min Limiters
  Sensor : Inport
  Alt : Inport  Port=2
  "Wfdmd " : Inport  Port=3
  Bus Selector1 : BusSelector  OutputSignals=P.Ps3sen
  Bus Selector11 : BusSelector  OutputSignals=P.Ps3sen
  Mux : Mux  Inputs=2
  Ps3 Limit : Subsystem
  Wf/Ps3 Limit : Subsystem
  Wfmn : Outport
  MnD : Outport  Port=2
  wires:
  Sensor/1 -> Bus Selector1/1, Bus Selector11/1
  Mux/1 -> Wfmn/1
  Bus Selector1/1 -> Wf/Ps3 Limit/1(Ps3)  "<Ps3sen>"
  Wf/Ps3 Limit/1(WfLim) -> Mux/2
  Alt/1 -> Ps3 Limit/1(Alt)
  Bus Selector11/1 -> Ps3 Limit/2(Ps3)  "<Ps3sen>"
  "Wfdmd "/1 -> Ps3 Limit/3(Wfdmd)
  Ps3 Limit/1(WfLim) -> Mux/1
  Ps3 Limit/2(Ps3Lim) -> MnD/1

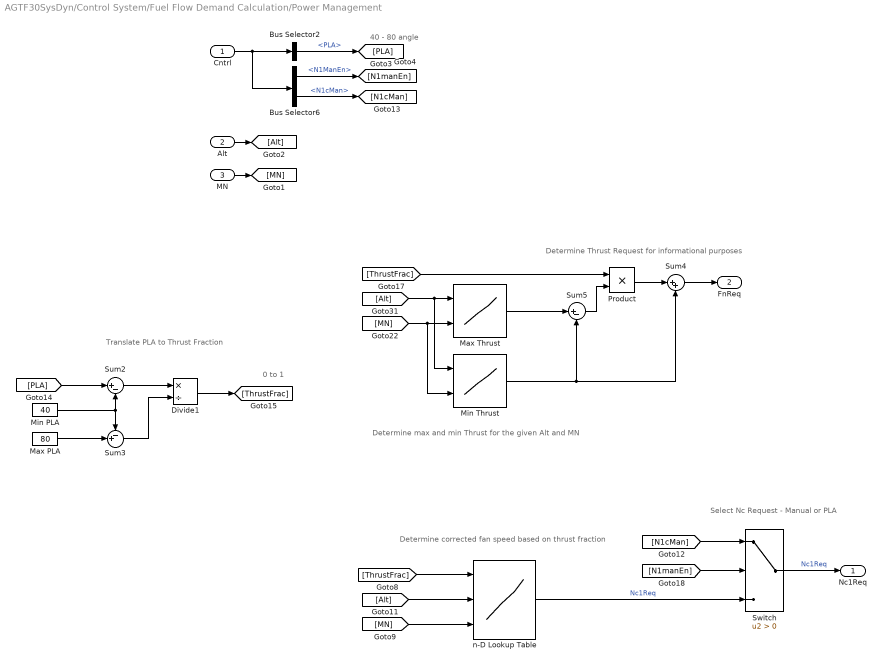
== system AGTF30SysDyn/Control System/Fuel Flow Demand Calculation/Power Management ==
  note: Determine corrected fan speed based on thrust fraction
  note: 0 to 1
  note: Determine max and min Thrust for the given Alt and MN
  note: 40 - 80 angle
  note: Translate PLA to Thrust Fraction
  note: Determine Thrust Request for informational purposes
  note: Select Nc Request - Manual or PLA
  Cntrl : Inport
  Alt : Inport  Port=2
  MN : Inport  Port=3
  Bus Selector2 : BusSelector  OutputSignals=PLA
  Bus Selector6 : BusSelector  OutputSignals=ManualOp.N1ManEn,ManualOp.N1cMan
  Divide1 : Product  Inputs=*/
  Max PLA : Constant  Value=80
  Max Thrust : Lookup_n-D  BreakpointsForDimension1=MWS.Cntrl.Fn_AltVec  BreakpointsForDimension2=MWS.Cntrl.Fn_MNVec  Table=MWS.Cntrl.Fn_mx  InternalRulePriority=Speed  RndMeth=Simplest  InputSameDT=on
  Min PLA : Constant  Value=40
  Min Thrust : Lookup_n-D  BreakpointsForDimension1=MWS.Cntrl.Fn_AltVec  BreakpointsForDimension2=MWS.Cntrl.Fn_MNVec  Table=MWS.Cntrl.Fn_mn  InternalRulePriority=Speed  RndMeth=Simplest  InputSameDT=on
  Product : Product
  Sum2 : Sum  Inputs=|+-
  Sum3 : Sum  Inputs=-+|
  Sum4 : Sum  Inputs=|++
  Sum5 : Sum  Inputs=|+-
  Switch : Switch  Criteria=u2 > Threshold
  n-D Lookup Table : Lookup_n-D  NumberOfTableDimensions=3  BreakpointsForDimension1=MWS.Cntrl.PM_TF  BreakpointsForDimension2=MWS.Cntrl.PM_AltVec  BreakpointsForDimension3=MWS.Cntrl.PM_MNVec  Table=MWS.Cntrl.PM_NcArray  InternalRulePriority=Speed  RndMeth=Simplest  InputSameDT=on
  Nc1Req : Outport
  FnReq : Outport  Port=2
  wires:
  Switch/1 -> Nc1Req/1  "Nc1Req"
  Bus Selector6/2 -> [N1cMan]  "<N1cMan>"
  Bus Selector6/1 -> [N1manEn]  "<N1ManEn>"
  Cntrl/1 -> Bus Selector6/1, Bus Selector2/1
  Bus Selector2/1 -> [PLA]  "<PLA>"
  Alt/1 -> [Alt]
  MN/1 -> [MN]
  [Alt] -> Min Thrust/1, Max Thrust/1
  [MN] -> Min Thrust/2, Max Thrust/2
  [PLA] -> Sum2/1
  Min PLA/1 -> Sum3/1, Sum2/2
  Max PLA/1 -> Sum3/2
  Sum2/1 -> Divide1/1
  Sum3/1 -> Divide1/2
  Divide1/1 -> [ThrustFrac]
  Max Thrust/1 -> Sum5/1
  [ThrustFrac] -> Product/1
  Min Thrust/1 -> Sum4/2, Sum5/2
  Sum5/1 -> Product/2
  Product/1 -> Sum4/1
  Sum4/1 -> FnReq/1
  [ThrustFrac] -> n-D Lookup Table/1
  [Alt] -> n-D Lookup Table/2
  [MN] -> n-D Lookup Table/3
  n-D Lookup Table/1 -> Switch/3  "Nc1Req"
  [N1manEn] -> Switch/2
  [N1cMan] -> Switch/1

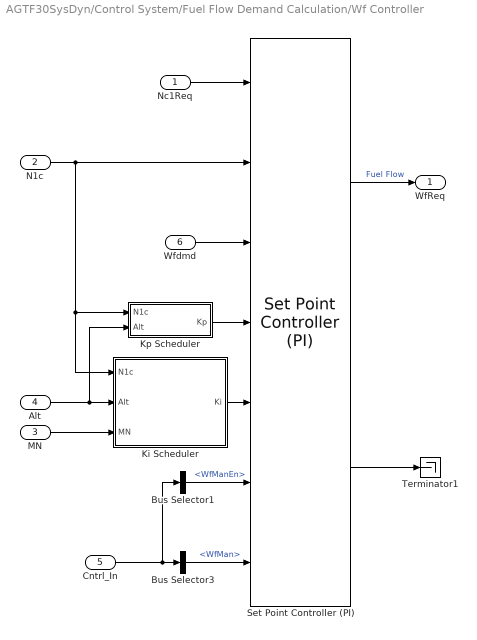
== system AGTF30SysDyn/Control System/Fuel Flow Demand Calculation/Wf Controller ==
  Nc1Req : Inport
  N1c : Inport  Port=2
  MN : Inport  Port=3
  Alt : Inport  Port=4
  Cntrl_In : Inport  Port=5
  Wfdmd : Inport  Port=6
  Bus Selector1 : BusSelector  OutputSignals=ManualOp.WfManEn
  Bus Selector3 : BusSelector  OutputSignals=ManualOp.WfMan
  Ki Scheduler : Subsystem
  Kp Scheduler : Subsystem
  Set Point Controller (PI) : Lib_Cntrl_SetPointCntrlPI_TMATS/Set Point Controller (PI)  PI_IC_M=MWS.In.WfIC  WGain_M=2000  Ts_M=MWS.In.Ts
  Terminator1 : Terminator
  WfReq : Outport
  wires:
  Wfdmd/1 -> Set Point Controller (PI)/3
  Set Point Controller (PI)/2 -> Terminator1/1
  Alt/1 -> Kp Scheduler/2(Alt), Ki Scheduler/2(Alt)
  MN/1 -> Ki Scheduler/3(MN)
  Bus Selector1/1 -> Set Point Controller (PI)/6  "<WfManEn>"
  Bus Selector3/1 -> Set Point Controller (PI)/7  "<WfMan>"
  Nc1Req/1 -> Set Point Controller (PI)/1
  Kp Scheduler/1(Kp) -> Set Point Controller (PI)/4
  Ki Scheduler/1(Ki) -> Set Point Controller (PI)/5
  Cntrl_In/1 -> Bus Selector1/1, Bus Selector3/1
  Set Point Controller (PI)/1 -> WfReq/1  "Fuel Flow"
  N1c/1 -> Ki Scheduler/1(N1c), Kp Scheduler/1(N1c), Set Point Controller (PI)/2

== system AGTF30SysDyn/Control System/Fuel Flow Demand Calculation/Max Limiters/N1 Limit ==
  N1 : Inport
  Wfdmd : Inport  Port=2
  N1 max limiter : Lib_Cntrl_LimitCntrlPI_TMATS/Limit Controller (PI)  Kp_M=MWS.Cntrl.N1mx_Kp  Ki_M=MWS.Cntrl.N1mx_Ki  PI_IC_M=MWS.In.WfIC  WGain_M=2000  Ts_M=MWS.In.Ts
  N1_limit : Constant  Value=MWS.Cntrl.N1_MAX
  Terminator1 : Terminator
  WfLim : Outport
  wires:
  N1 max limiter/1 -> WfLim/1
  N1 max limiter/2 -> Terminator1/1
  N1/1 -> N1 max limiter/2
  N1_limit/1 -> N1 max limiter/1
  Wfdmd/1 -> N1 max limiter/3

== system AGTF30SysDyn/Control System/Fuel Flow Demand Calculation/Max Limiters/N3 Limit ==
  N3 : Inport
  Wfdmd : Inport  Port=2
  N3 max limiter : Lib_Cntrl_LimitCntrlPI_TMATS/Limit Controller (PI)  Kp_M=MWS.Cntrl.N3mx_Kp  Ki_M=MWS.Cntrl.N3mx_Ki  PI_IC_M=MWS.In.WfIC  WGain_M=2000  Ts_M=MWS.In.Ts
  N3_limit : Constant  Value=MWS.Cntrl.N3_MAX
  Terminator4 : Terminator
  WfLim : Outport
  wires:
  N3_limit/1 -> N3 max limiter/1
  N3 max limiter/1 -> WfLim/1
  N3 max limiter/2 -> Terminator4/1
  N3/1 -> N3 max limiter/2
  Wfdmd/1 -> N3 max limiter/3

== system AGTF30SysDyn/Control System/Fuel Flow Demand Calculation/Max Limiters/Ps3 Limit ==
  Ps3 : Inport
  Wfdmd : Inport  Port=2
  Ps3 max limiter : Lib_Cntrl_LimitCntrlPI_TMATS/Limit Controller (PI)  Kp_M=MWS.Cntrl.Ps3mx_Kp  Ki_M=MWS.Cntrl.Ps3mx_Ki  PI_IC_M=MWS.In.WfIC  WGain_M=2000  Ts_M=MWS.In.Ts
  Ps3max_limit : Constant  Value=MWS.Cntrl.Ps3_MAX
  Terminator5 : Terminator
  WfLim : Outport
  wires:
  Ps3 max limiter/1 -> WfLim/1
  Ps3/1 -> Ps3 max limiter/2
  Ps3max_limit/1 -> Ps3 max limiter/1
  Ps3 max limiter/2 -> Terminator5/1
  Wfdmd/1 -> Ps3 max limiter/3

== system AGTF30SysDyn/Control System/Fuel Flow Demand Calculation/Max Limiters/T45 Limit ==
  MN : Inport
  Alt : Inport  Port=2
  T45 : Inport  Port=3
  Wfdmd : Inport  Port=4
  Constant2 : Constant  Value=0
  T45 limit definition : Subsystem
  T45 max limiter : Lib_Cntrl_LimitCntrlPI_TMATS/Limit Controller (PI)  Kp_M=MWS.Cntrl.T45mx_Kp  Ki_M=MWS.Cntrl.T45mx_Ki  PI_IC_M=MWS.In.WfIC  WGain_M=2000  Ts_M=MWS.In.Ts
  Terminator : Terminator
  WfLim : Outport
  T45Lim : Outport  Port=2
  wires:
  T45 max limiter/1 -> WfLim/1
  T45 max limiter/2 -> Terminator/1
  T45 limit definition/1(T45er) -> T45Lim/1, T45 max limiter/1
  T45/1 -> T45 limit definition/3(T45_sen)
  MN/1 -> T45 limit definition/1(MN)
  Alt/1 -> T45 limit definition/2(Alt)
  Constant2/1 -> T45 max limiter/2
  Wfdmd/1 -> T45 max limiter/3

== system AGTF30SysDyn/Control System/Fuel Flow Demand Calculation/Max Limiters/Wf/Ps3 Limit ==
  N1c : Inport
  Alt : Inport  Port=2
  Ps3 : Inport  Port=3
  1-D Lookup Table1 : Lookup_n-D  NumberOfTableDimensions=1  BreakpointsForDimension1=MWS.Cntrl.RU_Nc  Table=MWS.Cntrl.RUmx  InternalRulePriority=Speed  RndMeth=Simplest  InputSameDT=on
  N1_limit1 : Constant  Value=1/40000
  N1_limit2 : Constant  Value=300
  Product : Product
  Product1 : Product  Inputs=3
  Sum : Sum  Inputs=|+-
  WfLim : Outport
  WfqPs3Lim : Outport  Port=2
  wires:
  Ps3/1 -> Product/2
  N1_limit1/1 -> Product1/3
  Alt/1 -> Product1/1
  1-D Lookup Table1/1 -> WfqPs3Lim/1, Product/1
  Sum/1 -> 1-D Lookup Table1/1
  Product/1 -> WfLim/1
  N1c/1 -> Sum/1
  N1_limit2/1 -> Product1/2
  Product1/1 -> Sum/2

== system AGTF30SysDyn/Control System/Fuel Flow Demand Calculation/Min Limiters/Ps3 Limit ==
  Alt : Inport
  Ps3 : Inport  Port=2
  Wfdmd : Inport  Port=3
  1-D Lookup Table : Lookup_n-D  NumberOfTableDimensions=1  BreakpointsForDimension1=MWS.Cntrl.Ps3mn_AltVec  Table=MWS.Cntrl.Ps3mn_Ps3Lim  InternalRulePriority=Speed  RndMeth=Simplest  InputSameDT=on
  Ps3sen : Lib_Cntrl_LimitCntrlPI_TMATS/Limit Controller (PI)  Kp_M=MWS.Cntrl.Ps3mn_Kp  Ki_M=MWS.Cntrl.Ps3mn_Ki  PI_IC_M=MWS.In.WfIC  WGain_M=2000  Ts_M=MWS.In.Ts
  Terminator2 : Terminator
  WfLim : Outport
  Ps3Lim : Outport  Port=2
  wires:
  Ps3/1 -> Ps3sen/2
  1-D Lookup Table/1 -> Ps3sen/1, Ps3Lim/1
  Ps3sen/1 -> WfLim/1
  Wfdmd/1 -> Ps3sen/3
  Ps3sen/2 -> Terminator2/1
  Alt/1 -> 1-D Lookup Table/1

== system AGTF30SysDyn/Control System/Fuel Flow Demand Calculation/Min Limiters/Wf/Ps3 Limit ==
  Ps3 : Inport
  N1_limit2 : Constant  Value=MWS.Cntrl.RUmn
  Product : Product
  WfLim : Outport
  wires:
  Ps3/1 -> Product/1
  N1_limit2/1 -> Product/2
  Product/1 -> WfLim/1

== system AGTF30SysDyn/Control System/Fuel Flow Demand Calculation/Wf Controller/Ki Scheduler ==
  N1c : Inport
  Alt : Inport  Port=2
  MN : Inport  Port=3
  GainLookupK1 : Lookup_n-D  BreakpointsForDimension1=MWS.Cntrl.Ki_NcVec  BreakpointsForDimension2=MWS.Cntrl.Ki_AltVec  Table=MWS.Cntrl.Ki_sch'  InterpMethod=Nearest  DiagnosticForOutOfRangeInput=Warning  InternalRulePriority=Speed  RndMeth=Simplest  InputSameDT=on
  GainLookupK2 : Lookup_n-D  BreakpointsForDimension1=MWS.Cntrl.Ki_MNVecX  BreakpointsForDimension2=MWS.Cntrl.Ki_AltVecX  Table=MWS.Cntrl.KiX_sch'  InterpMethod=Flat  DiagnosticForOutOfRangeInput=Warning  InternalRulePriority=Speed  RndMeth=Simplest  InputSameDT=on
  Mux1 : Mux  Inputs=2
  Ki : Outport
  wires:
  N1c/1 -> GainLookupK1/1
  Alt/1 -> GainLookupK1/2, GainLookupK2/2
  Mux1/1 -> Ki/1
  GainLookupK2/1 -> Mux1/2
  GainLookupK1/1 -> Mux1/1
  MN/1 -> GainLookupK2/1

== system AGTF30SysDyn/Control System/Fuel Flow Demand Calculation/Wf Controller/Kp Scheduler ==
  N1c : Inport
  Alt : Inport  Port=2
  GainLookupK1 : Lookup_n-D  BreakpointsForDimension1=MWS.Cntrl.Kp_NcVec  BreakpointsForDimension2=MWS.Cntrl.Kp_AltVec  Table=MWS.Cntrl.Kp_sch'  InterpMethod=Nearest  DiagnosticForOutOfRangeInput=Warning  InternalRulePriority=Speed  RndMeth=Simplest  InputSameDT=on
  Kp : Outport
  wires:
  GainLookupK1/1 -> Kp/1
  N1c/1 -> GainLookupK1/1
  Alt/1 -> GainLookupK1/2

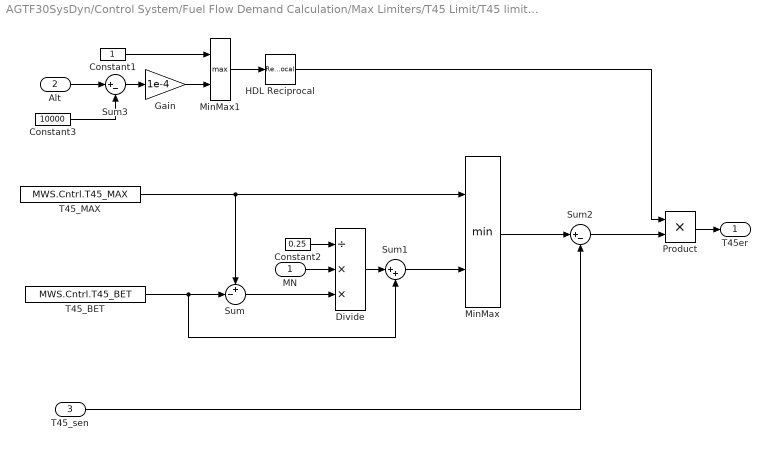
== system AGTF30SysDyn/Control System/Fuel Flow Demand Calculation/Max Limiters/T45 Limit/T45 limit definition ==
  MN : Inport
  Alt : Inport  Port=2
  T45_sen : Inport  Port=3
  Constant1 : Constant
  Constant2 : Constant  Value=0.25
  Constant3 : Constant  Value=10000
  Divide : Product  Inputs=/**
  Gain : Gain  Gain=1e-4
  HDL Reciprocal : Reciprocal
  MinMax : MinMax  Inputs=2
  MinMax1 : MinMax  Function=max  Inputs=2
  Product : Product
  Sum : Sum  Inputs=+-|
  Sum1 : Sum  Inputs=|++
  Sum2 : Sum  Inputs=|+-
  Sum3 : Sum  Inputs=|+-
  T45_BET : Constant  Value=MWS.Cntrl.T45_BET
  T45_MAX : Constant  Value=MWS.Cntrl.T45_MAX
  T45er : Outport
  wires:
  MN/1 -> Divide/2
  MinMax/1 -> Sum2/1
  T45_MAX/1 -> Sum/1, MinMax/1
  T45_BET/1 -> Sum1/2, Sum/2
  Sum/1 -> Divide/3
  Constant2/1 -> Divide/1
  Divide/1 -> Sum1/1
  Sum1/1 -> MinMax/2
  T45_sen/1 -> Sum2/2
  Product/1 -> T45er/1
  Sum2/1 -> Product/2
  Alt/1 -> Sum3/1
  Sum3/1 -> Gain/1
  Constant1/1 -> MinMax1/1
  Constant3/1 -> Sum3/2
  Gain/1 -> MinMax1/2
  MinMax1/1 -> HDL Reciprocal/1
  HDL Reciprocal/1 -> Product/1
